simulink subsystem "Motor_circuit"  (R2020b)
settings: Solver=VariableStepAuto  StartTime=0.0  StopTime=10.0  RelTol=1e-3
settings Model: Creator=avina  LastModifiedBy=avina

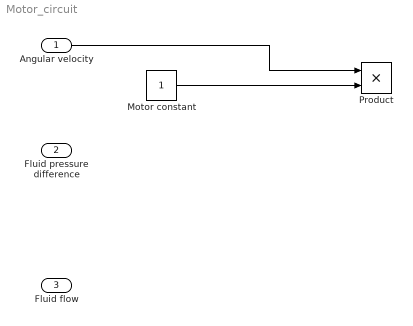
== system Motor_circuit ==
  Angular velocity : Inport
  Fluid pressure difference : Inport  Port=2
  Fluid flow : Inport  Port=3
  Motor constant : Constant
  Product : Product
  wires:
  Angular velocity/1 -> Product/1
  Motor constant/1 -> Product/2
